simulink library "lib_flux_observer"  (R2023a)
settings: Solver=VariableStepAuto  StartTime=0.0  StopTime=10.0  RelTol=1e-3
undefined symbols (not defined in the file): bit, parDirIndc_u16p29b0, parFluxObsFiltCoef, parMedTaskSampTime_u16d6b0, parPhsCurrMaxVal, parPhsRstnMaxVal, parPhsVoltMaxVal, parPolePairNum_u8n0b0
libraries: lib_conversion x13, lib_trigonometric_function x2, lib_iir_filter x2, lib_discrete_time_integrator x2, lib_cart_to_polar_coor_transformer x1
settings Model: Creator=cav2ofo  LastModifiedBy=lenovo
settings OptimizationCC: ReuseModelBlockBuffer=off

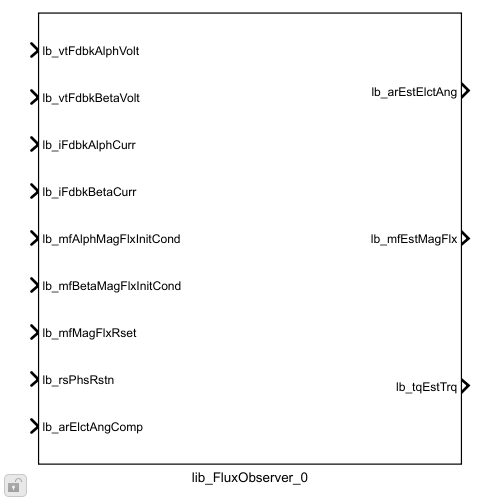
[thumbnail: Simulink's stored preview of the top-level diagram]
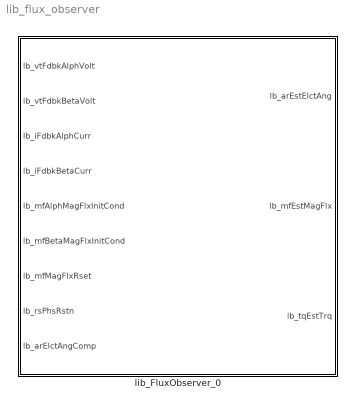
== system lib_flux_observer ==
  lib_FluxObserver_0 : Subsystem  mask{lb_parPhsIndc=parDirIndc_u16p29b0, lb_parPhsRstnMaxVal=parPhsRstnMaxVal, lb_parPhsIndcMaxVal=parPhsRstnMaxVal, lb_parPhsCurrMaxVal=parPhsCurrMaxVal, lb_parPhsVoltMaxVal=parPhsVoltMaxVal, lb_parEstMagFluxMaxVal=0.01, lb_parPolePairNum=parPolePairNum_u8n0b0, lb_parSampTime=parMedTaskSampTime_u16d6b0, lb_parFltrCoefMaxVal=double(parFluxObsFiltCoef), lb_parFiltCoef=parFluxObsFiltCoef, lb_parFluxDataType=fixdt(0,16,2^-22,0), lb_parMotTrqDataType=fixdt(1,16,2^-14,0), lb_parBitNumMode=32-bit}
      mask prompts: lb_parPhsIndc "Phase inductance [H]:"; lb_parPhsRstnMaxVal "Maximum phase resistance [Ohm]:"; lb_parPhsIndcMaxVal "Maximum phase inductance [H]:"; lb_parPhsCurrMaxVal "Maximum phase current [A]:"; lb_parPhsVoltMaxVal "Maximum phase voltage [V]:"; lb_parEstMagFluxMaxVal "Maximum estimated magnet flux [Wb]:"; lb_parPolePairNum "Number of pole pairs:"; lb_parSampTime "Sampling time [s]:"; lb_parFltrCoefMaxVal "High-pass filter coefficient max value:"; lb_parFiltCoef "High-pass filter coefficient:"; lb_parFluxDataType "Permanent magnet flux data type:"; lb_parMotTrqDataType "Motor electric torque data type:"; lb_parBitNumMode "Bits number for internal calculations:"
      mask init:
      | switch lb_parBitNumMode
      |     case '16-bit'
      |         lb_parBitNum = 16;
      |     case '32-bit'
      |         lb_parBitNum = 32;
      |     otherwise
      |         lb_parBitNum = 16;
      | end
      | 
      | % Operation 1: R*I
      | lb_parOper1MaxVal = lb_parPhsRstnMaxVal*lb_parPhsCurrMaxVal;
      | 
      | % Operation 2: V-R*I
      | lb_parOper2MaxVal = lb_parPhsVoltMaxVal+lb_parPhsRstnMaxVal*lb_parPhsCurrMaxVal;
      | 
      | % Operation 3: L*I
      | lb_parOper3MaxVal = lb_parPhsIndcMaxVal*lb_parPhsCurrMaxVal;
      | 
      | % Operation 4: integral of V-R*I
      | temp.intgMaxVal = lb_parOper3MaxVal+lb_parEstMagFluxMaxVal;
      | temp.NumType = fi(temp.intgMaxVal,1,lb_parBitNum);
      | lb_parIntgSlopExp = temp.NumType.FractionLength;
      | 
      | % Operation 5: filtering of flux
      | temp.NumType = fi(lb_parEstMagFluxMaxVal,1,16);
      | lb_parFiltSlopExp = temp.NumType.FractionLength;
      | 
      | % Operation 6: psi*I
      | lb_parOper6MaxVal = lb_parPhsCurrMaxVal*lb_parEstMagFluxMaxVal;
      | 
      | % Operation 7: 2*psi*I
      | lb_parOper7MaxVal = 2*lb_parPhsCurrMaxVal*lb_parEstMagFluxMaxVal;
      | 
      | % Operation 8: 3/2*Np
      | lb_parOper8MaxVal = 3/2*double(lb_parPolePairNum);
      mask TypeOptions lb_parFltrCoefMaxVal: sss_FluxAlphaBetaEstimation/lib_IirFilter_1/lb_parFltrCoefMaxVal | sss_FluxAlphaBetaEstimation/lib_IirFilter_2/lb_parFltrCoefMaxVal
      mask TypeOptions lb_parBitNumMode: 16-bit | 32-bit
      mask DialogControl DescGroupVar Prompt: Current Coupling block
      mask DialogControl DescTextVar Prompt: This block estimates electric angle, Permenant magnet flux and electric torque
      mask DialogControl modlPar Prompt: Model Parameters
      mask DialogControl Container3_copy Prompt: Data type:
      mask DialogControl Container3 Prompt: Operating modes:

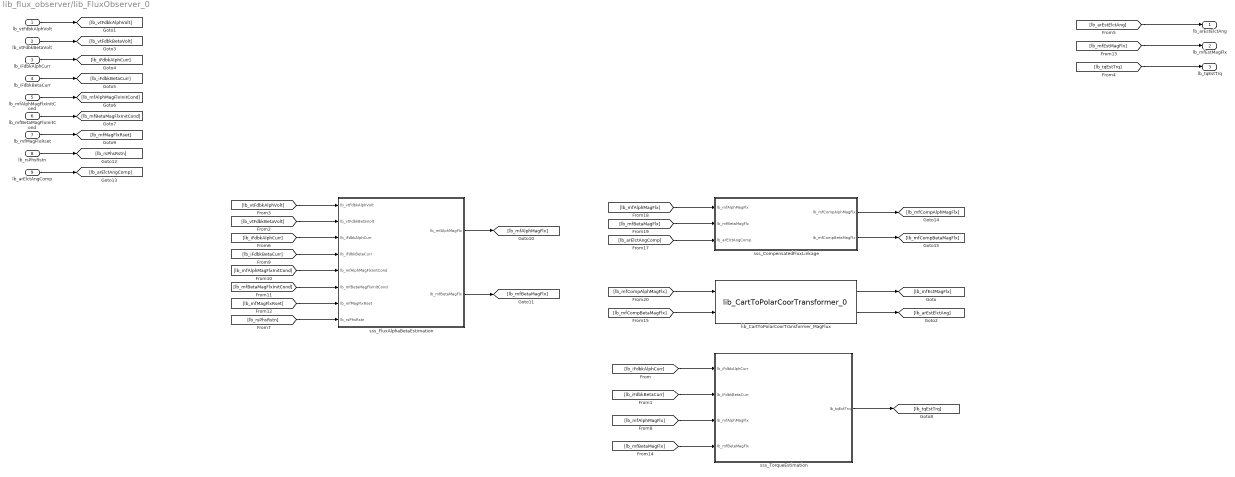
== system lib_flux_observer/lib_FluxObserver_0 ==
  lb_vtFdbkAlphVolt : Inport
  lb_vtFdbkBetaVolt : Inport  Port=2
  lb_iFdbkAlphCurr : Inport  Port=3
  lb_iFdbkBetaCurr : Inport  Port=4
  lb_mfAlphMagFlxInitCond : Inport  Port=5
  lb_mfBetaMagFlxInitCond : Inport  Port=6
  lb_mfMagFlxRset : Inport  Port=7
  lb_rsPhsRstn : Inport  Port=8
  lb_arElctAngComp : Inport  Port=9  OutDataTypeStr=fixdt(0,16,pi*2^-15,0)
  lib_CartToPolarCoorTransformer_MagFlux : lib_cart_to_polar_coor_transformer/lib_CartToPolarCoorTransformer_0  lb_parAsinLktSize=4095  lb_parAmpLktSize=512  lb_parOutpAmpDataType=lb_parFluxDataType
  sss_CompensatedFluxLinkage : Subsystem
  sss_FluxAlphaBetaEstimation : Subsystem
  sss_TorqueEstimation : Subsystem
  lb_arEstElctAng : Outport
  lb_mfEstMagFlx : Outport  Port=2
  lb_tqEstTrq : Outport  Port=3
  wires:
  sss_CompensatedFluxLinkage/2(lb_mfCompBetaMagFlx) -> [lb_mfCompBetaMagFlx]
  sss_CompensatedFluxLinkage/1(lb_mfCompAlphMagFlx) -> [lb_mfCompAlphMagFlx]
  [lb_mfBetaMagFlx] -> sss_CompensatedFluxLinkage/2(lb_mfBetaMagFlx)
  [lb_mfAlphMagFlx] -> sss_CompensatedFluxLinkage/1(lb_mfAlphMagFlx)
  [lb_arElctAngComp] -> sss_CompensatedFluxLinkage/3(lb_arElctAngComp)
  lb_arElctAngComp/1 -> [lb_arElctAngComp]
  [lb_rsPhsRstn] -> sss_FluxAlphaBetaEstimation/8(lb_rsPhsRstn)
  lb_rsPhsRstn/1 -> [lb_rsPhsRstn]
  [lb_mfCompAlphMagFlx] -> lib_CartToPolarCoorTransformer_MagFlux/1
  [lb_mfCompBetaMagFlx] -> lib_CartToPolarCoorTransformer_MagFlux/2
  lib_CartToPolarCoorTransformer_MagFlux/2 -> [lb_arEstElctAng]
  [lb_tqEstTrq] -> lb_tqEstTrq/1
  [lb_iFdbkBetaCurr] -> sss_TorqueEstimation/2(lb_iFdbkBetaCurr)
  [lb_iFdbkAlphCurr] -> sss_TorqueEstimation/1(lb_iFdbkAlphCurr)
  [lb_mfBetaMagFlx] -> sss_TorqueEstimation/4(lb_mfBetaMagFlx)
  [lb_mfAlphMagFlx] -> sss_TorqueEstimation/3(lb_mfAlphMagFlx)
  sss_FluxAlphaBetaEstimation/2(lb_mfBetaMagFlx) -> [lb_mfBetaMagFlx]
  sss_FluxAlphaBetaEstimation/1(lb_mfAlphMagFlx) -> [lb_mfAlphMagFlx]
  [lb_mfMagFlxRset] -> sss_FluxAlphaBetaEstimation/7(lb_mfMagFlxRset)
  lb_mfMagFlxRset/1 -> [lb_mfMagFlxRset]
  [lb_mfBetaMagFlxInitCond] -> sss_FluxAlphaBetaEstimation/6(lb_mfBetaMagFlxInitCond)
  [lb_mfAlphMagFlxInitCond] -> sss_FluxAlphaBetaEstimation/5(lb_mfAlphMagFlxInitCond)
  lb_mfAlphMagFlxInitCond/1 -> [lb_mfAlphMagFlxInitCond]
  lb_mfBetaMagFlxInitCond/1 -> [lb_mfBetaMagFlxInitCond]
  [lb_iFdbkBetaCurr] -> sss_FluxAlphaBetaEstimation/4(lb_iFdbkBetaCurr)
  [lb_vtFdbkBetaVolt] -> sss_FluxAlphaBetaEstimation/2(lb_vtFdbkBetaVolt)
  [lb_vtFdbkAlphVolt] -> sss_FluxAlphaBetaEstimation/1(lb_vtFdbkAlphVolt)
  lib_CartToPolarCoorTransformer_MagFlux/1 -> [lb_mfEstMagFlx]
  [lb_arEstElctAng] -> lb_arEstElctAng/1
  [lb_iFdbkAlphCurr] -> sss_FluxAlphaBetaEstimation/3(lb_iFdbkAlphCurr)
  lb_iFdbkAlphCurr/1 -> [lb_iFdbkAlphCurr]
  lb_vtFdbkBetaVolt/1 -> [lb_vtFdbkBetaVolt]
  sss_TorqueEstimation/1(lb_tqEstTrq) -> [lb_tqEstTrq]
  [lb_mfEstMagFlx] -> lb_mfEstMagFlx/1
  lb_iFdbkBetaCurr/1 -> [lb_iFdbkBetaCurr]
  lb_vtFdbkAlphVolt/1 -> [lb_vtFdbkAlphVolt]

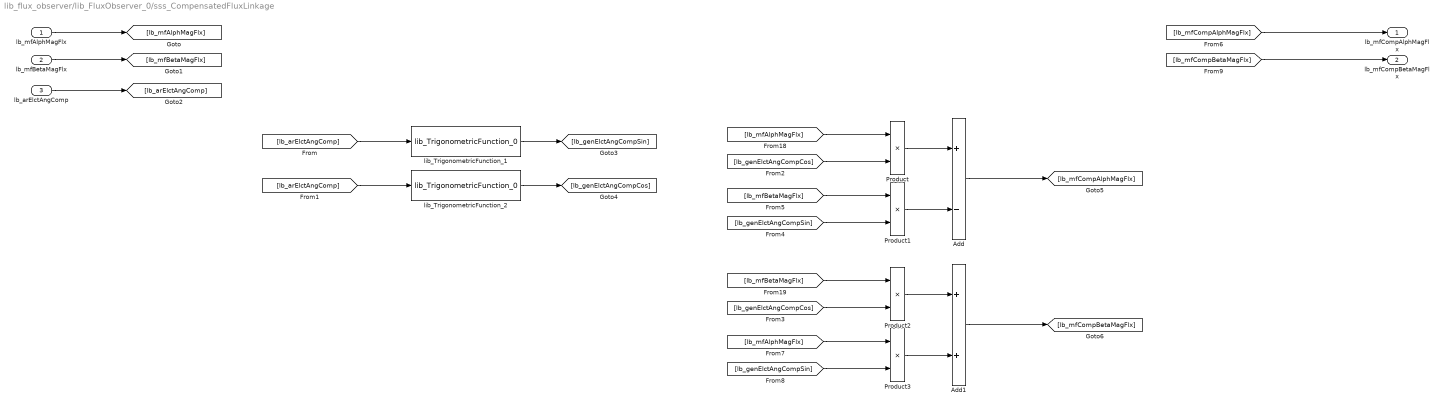
== system lib_flux_observer/lib_FluxObserver_0/sss_CompensatedFluxLinkage ==
  lb_mfAlphMagFlx : Inport
  lb_mfBetaMagFlx : Inport  Port=2
  lb_arElctAngComp : Inport  Port=3
  Add : Sum  Inputs=+-  OutDataTypeStr=Inherit: Same as first input
  Add1 : Sum  OutDataTypeStr=Inherit: Same as first input
  Product{,1..3} (4 alike) : Product  OutDataTypeStr=Inherit: Same as first input
  lib_TrigonometricFunction_1 : lib_trigonometric_function/lib_TrigonometricFunction_0  lb_parSelSigType=Sine  lb_parLktSizeStr=1024  lb_parOutpDataType=fixdt(1,16,2^-14,0)
  lib_TrigonometricFunction_2 : lib_trigonometric_function/lib_TrigonometricFunction_0  lb_parSelSigType=Cosine  lb_parLktSizeStr=1024  lb_parOutpDataType=fixdt(1,16,2^-14,0)
  lb_mfCompAlphMagFlx : Outport
  lb_mfCompBetaMagFlx : Outport  Port=2
  wires:
  [lb_mfCompBetaMagFlx] -> lb_mfCompBetaMagFlx/1
  [lb_mfCompAlphMagFlx] -> lb_mfCompAlphMagFlx/1
  Product2/1 -> Add1/1
  [lb_mfBetaMagFlx] -> Product2/1
  Product3/1 -> Add1/2
  Add1/1 -> [lb_mfCompBetaMagFlx]
  [lb_genElctAngCompSin] -> Product3/2
  [lb_genElctAngCompCos] -> Product2/2
  [lb_mfAlphMagFlx] -> Product3/1
  Add/1 -> [lb_mfCompAlphMagFlx]
  Product/1 -> Add/1
  Product1/1 -> Add/2
  [lb_mfBetaMagFlx] -> Product1/1
  [lb_genElctAngCompSin] -> Product1/2
  [lb_genElctAngCompCos] -> Product/2
  [lb_mfAlphMagFlx] -> Product/1
  lib_TrigonometricFunction_2/1 -> [lb_genElctAngCompCos]
  lib_TrigonometricFunction_1/1 -> [lb_genElctAngCompSin]
  [lb_arElctAngComp] -> lib_TrigonometricFunction_2/1
  [lb_arElctAngComp] -> lib_TrigonometricFunction_1/1
  lb_arElctAngComp/1 -> [lb_arElctAngComp]
  lb_mfBetaMagFlx/1 -> [lb_mfBetaMagFlx]
  lb_mfAlphMagFlx/1 -> [lb_mfAlphMagFlx]

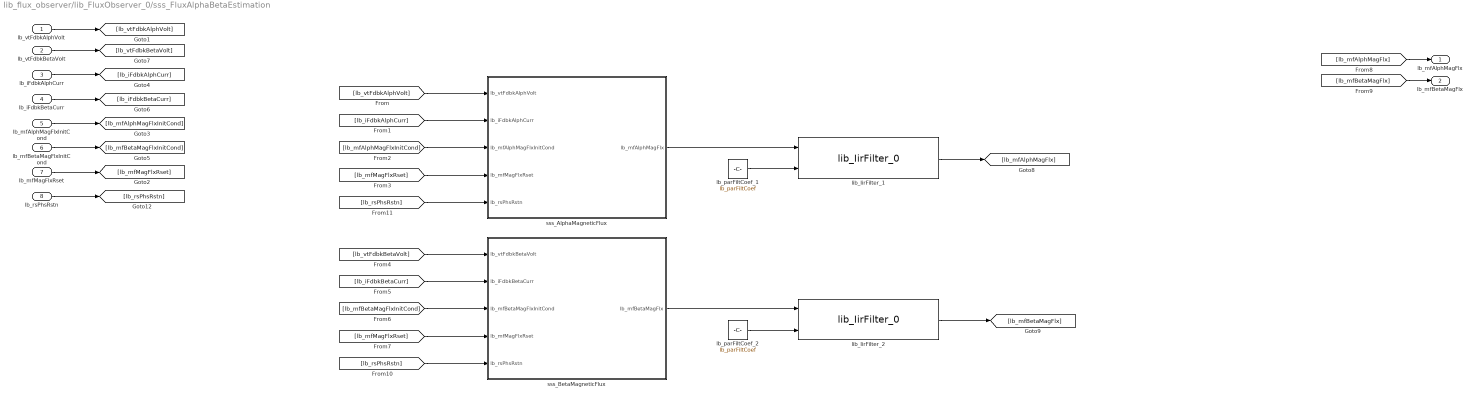
== system lib_flux_observer/lib_FluxObserver_0/sss_FluxAlphaBetaEstimation ==
  lb_vtFdbkAlphVolt : Inport
  lb_vtFdbkBetaVolt : Inport  Port=2
  lb_iFdbkAlphCurr : Inport  Port=3
  lb_iFdbkBetaCurr : Inport  Port=4
  lb_mfAlphMagFlxInitCond : Inport  Port=5
  lb_mfBetaMagFlxInitCond : Inport  Port=6
  lb_mfMagFlxRset : Inport  Port=7
  lb_rsPhsRstn : Inport  Port=8
  lb_parFiltCoef_1 : Constant  Value=lb_parFiltCoef
  lb_parFiltCoef_2 : Constant  Value=lb_parFiltCoef
  lib_IirFilter_1 : lib_iir_filter/lib_IirFilter_0  lb_parMaxInpVal=lb_parEstMagFluxMaxVal  lb_parFltrCoefMaxVal=lb_parFltrCoefMaxVal  lb_parBitNumMode=32-bit  lb_parOutpDataType=fixdt(1,16,2^-lb_parFiltSlopExp,0)  lb_parFiltTypeMode=High-pass
      link override vss_FilterVariant: VariantControlMode=label  LabelModeActiveChoice=lb_parHighPassModeLbl
  lib_IirFilter_2 : lib_iir_filter/lib_IirFilter_0  lb_parMaxInpVal=lb_parEstMagFluxMaxVal  lb_parFltrCoefMaxVal=lb_parFltrCoefMaxVal  lb_parBitNumMode=32-bit  lb_parOutpDataType=fixdt(1,16,2^-lb_parFiltSlopExp,0)  lb_parFiltTypeMode=High-pass
      link override vss_FilterVariant: VariantControlMode=label  LabelModeActiveChoice=lb_parHighPassModeLbl
  sss_AlphaMagneticFlux : Subsystem
  sss_BetaMagneticFlux : Subsystem
  lb_mfAlphMagFlx : Outport
  lb_mfBetaMagFlx : Outport  Port=2
  wires:
  lib_IirFilter_2/1 -> [lb_mfBetaMagFlx]
  lb_parFiltCoef_2/1 -> lib_IirFilter_2/2
  lb_parFiltCoef_1/1 -> lib_IirFilter_1/2
  sss_BetaMagneticFlux/1(lb_mfBetaMagFlx) -> lib_IirFilter_2/1
  [lb_rsPhsRstn] -> sss_AlphaMagneticFlux/5(lb_rsPhsRstn)
  [lb_rsPhsRstn] -> sss_BetaMagneticFlux/5(lb_rsPhsRstn)
  lb_rsPhsRstn/1 -> [lb_rsPhsRstn]
  lib_IirFilter_1/1 -> [lb_mfAlphMagFlx]
  sss_AlphaMagneticFlux/1(lb_mfAlphMagFlx) -> lib_IirFilter_1/1
  [lb_mfBetaMagFlx] -> lb_mfBetaMagFlx/1
  [lb_mfAlphMagFlx] -> lb_mfAlphMagFlx/1
  lb_vtFdbkBetaVolt/1 -> [lb_vtFdbkBetaVolt]
  lb_iFdbkBetaCurr/1 -> [lb_iFdbkBetaCurr]
  [lb_mfMagFlxRset] -> sss_BetaMagneticFlux/4(lb_mfMagFlxRset)
  [lb_vtFdbkBetaVolt] -> sss_BetaMagneticFlux/1(lb_vtFdbkBetaVolt)
  [lb_iFdbkBetaCurr] -> sss_BetaMagneticFlux/2(lb_iFdbkBetaCurr)
  [lb_mfBetaMagFlxInitCond] -> sss_BetaMagneticFlux/3(lb_mfBetaMagFlxInitCond)
  [lb_mfMagFlxRset] -> sss_AlphaMagneticFlux/4(lb_mfMagFlxRset)
  [lb_mfAlphMagFlxInitCond] -> sss_AlphaMagneticFlux/3(lb_mfAlphMagFlxInitCond)
  [lb_iFdbkAlphCurr] -> sss_AlphaMagneticFlux/2(lb_iFdbkAlphCurr)
  [lb_vtFdbkAlphVolt] -> sss_AlphaMagneticFlux/1(lb_vtFdbkAlphVolt)
  lb_mfBetaMagFlxInitCond/1 -> [lb_mfBetaMagFlxInitCond]
  lb_mfMagFlxRset/1 -> [lb_mfMagFlxRset]
  lb_vtFdbkAlphVolt/1 -> [lb_vtFdbkAlphVolt]
  lb_mfAlphMagFlxInitCond/1 -> [lb_mfAlphMagFlxInitCond]
  lb_iFdbkAlphCurr/1 -> [lb_iFdbkAlphCurr]

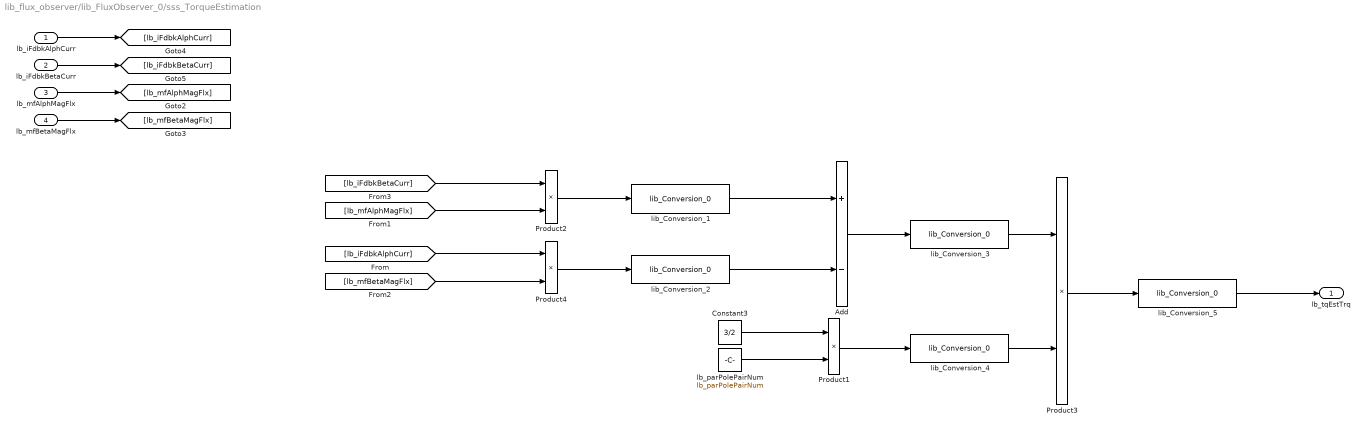
== system lib_flux_observer/lib_FluxObserver_0/sss_TorqueEstimation ==
  lb_iFdbkAlphCurr : Inport
  lb_iFdbkBetaCurr : Inport  Port=2
  lb_mfAlphMagFlx : Inport  Port=3
  lb_mfBetaMagFlx : Inport  Port=4
  Add : Sum  Inputs=+-  OutDataTypeStr=Inherit: Inherit via back propagation
  Constant3 : Constant  Value=3/2  OutDataTypeStr=fixdt(0,16,2^-15,0)
  Product{1..4} (4 alike) : Product  OutDataTypeStr=Inherit: Inherit via back propagation
  lb_parPolePairNum : Constant  Value=lb_parPolePairNum
  lib_Conversion_1 : lib_conversion/lib_Conversion_0  lb_parDataType=fixdt(1,16)  lb_parOutpMaxVal=lb_parOper6MaxVal  lb_parOutpMinVal=-lb_parOper6MaxVal  lb_parSatFlag=off
  lib_Conversion_2 : lib_conversion/lib_Conversion_0  lb_parDataType=fixdt(1,16)  lb_parOutpMaxVal=lb_parOper6MaxVal  lb_parOutpMinVal=-lb_parOper6MaxVal  lb_parSatFlag=off
  lib_Conversion_3 : lib_conversion/lib_Conversion_0  lb_parDataType=fixdt(1,16)  lb_parOutpMaxVal=lb_parOper7MaxVal  lb_parOutpMinVal=-lb_parOper7MaxVal  lb_parSatFlag=off
  lib_Conversion_4 : lib_conversion/lib_Conversion_0  lb_parDataType=fixdt(0,16)  lb_parOutpMaxVal=lb_parOper8MaxVal  lb_parOutpMinVal=[]  lb_parSatFlag=off
  lib_Conversion_5 : lib_conversion/lib_Conversion_0  lb_parDataType=lb_parMotTrqDataType  lb_parOutpMaxVal=[]  lb_parOutpMinVal=[]  lb_parSatFlag=off
  lb_tqEstTrq : Outport
  wires:
  lib_Conversion_2/1 -> Add/2
  Product4/1 -> lib_Conversion_2/1
  lib_Conversion_3/1 -> Product3/1
  lib_Conversion_4/1 -> Product3/2
  Product2/1 -> lib_Conversion_1/1
  lib_Conversion_1/1 -> Add/1
  Product1/1 -> lib_Conversion_4/1
  [lb_iFdbkBetaCurr] -> Product2/1
  [lb_mfAlphMagFlx] -> Product2/2
  [lb_iFdbkAlphCurr] -> Product4/1
  lb_iFdbkBetaCurr/1 -> [lb_iFdbkBetaCurr]
  lb_iFdbkAlphCurr/1 -> [lb_iFdbkAlphCurr]
  lb_parPolePairNum/1 -> Product1/2
  Constant3/1 -> Product1/1
  Add/1 -> lib_Conversion_3/1
  [lb_mfBetaMagFlx] -> Product4/2
  lib_Conversion_5/1 -> lb_tqEstTrq/1
  lb_mfBetaMagFlx/1 -> [lb_mfBetaMagFlx]
  lb_mfAlphMagFlx/1 -> [lb_mfAlphMagFlx]
  Product3/1 -> lib_Conversion_5/1

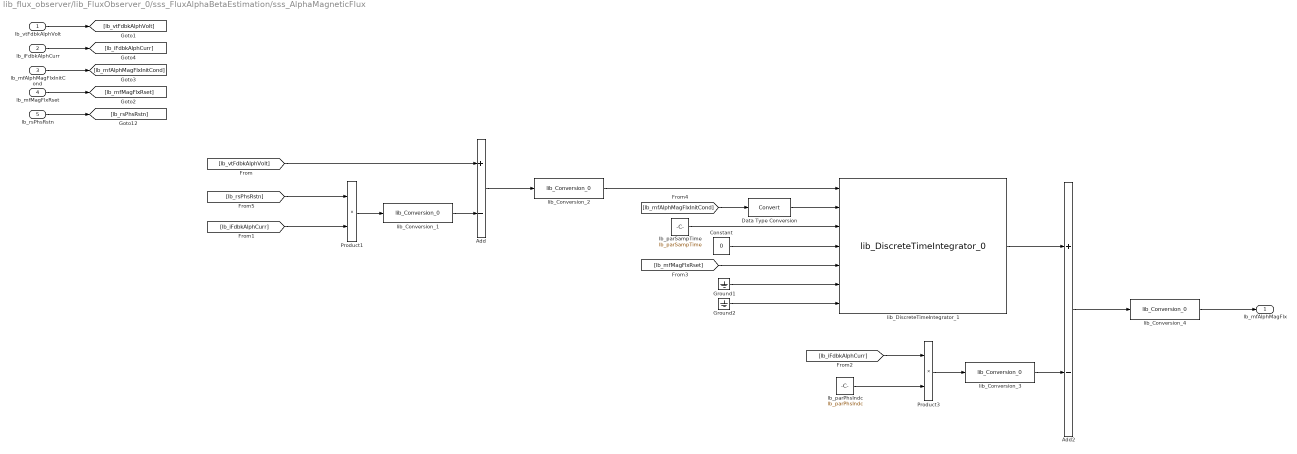
== system lib_flux_observer/lib_FluxObserver_0/sss_FluxAlphaBetaEstimation/sss_AlphaMagneticFlux ==
  lb_vtFdbkAlphVolt : Inport
  lb_iFdbkAlphCurr : Inport  Port=2
  lb_mfAlphMagFlxInitCond : Inport  Port=3
  lb_mfMagFlxRset : Inport  Port=4
  lb_rsPhsRstn : Inport  Port=5
  Add : Sum  Inputs=+-  OutDataTypeStr=Inherit: Inherit via back propagation
  Add2 : Sum  Inputs=+-  OutDataTypeStr=Inherit: Inherit via back propagation
  Constant : Constant  Value=0  OutDataTypeStr=uint8
  Data Type Conversion : DataTypeConversion  SaturateOnIntegerOverflow=off  RndMeth=Floor
  Ground1 : Ground
  Ground2 : Ground
  Product1 : Product  OutDataTypeStr=Inherit: Inherit via back propagation
  Product3 : Product  OutDataTypeStr=Inherit: Inherit via back propagation
  lb_parPhsIndc : Constant  Value=lb_parPhsIndc
  lb_parSampTime : Constant  Value=lb_parSampTime
  lib_Conversion_1 : lib_conversion/lib_Conversion_0  lb_parDataType=fixdt(1,lb_parBitNum)  lb_parOutpMaxVal=lb_parOper1MaxVal  lb_parOutpMinVal=-lb_parOper1MaxVal  lb_parSatFlag=off
  lib_Conversion_2 : lib_conversion/lib_Conversion_0  lb_parDataType=fixdt(1,lb_parBitNum)  lb_parOutpMaxVal=lb_parOper2MaxVal  lb_parOutpMinVal=-lb_parOper2MaxVal  lb_parSatFlag=off
  lib_Conversion_3 : lib_conversion/lib_Conversion_0  lb_parDataType=fixdt(1,lb_parBitNum)  lb_parOutpMaxVal=lb_parOper3MaxVal  lb_parOutpMinVal=-lb_parOper3MaxVal  lb_parSatFlag=off
  lib_Conversion_4 : lib_conversion/lib_Conversion_0  lb_parDataType=fixdt(1,lb_parBitNum)  lb_parOutpMaxVal=lb_parEstMagFluxMaxVal  lb_parOutpMinVal=-lb_parEstMagFluxMaxVal  lb_parSatFlag=off
  lib_DiscreteTimeIntegrator_1 : lib_discrete_time_integrator/lib_DiscreteTimeIntegrator_0  lb_parMaxInpVal=lb_parOper2MaxVal  lb_parMinInpVal=-lb_parOper2MaxVal  lb_parMaxSampTime=double(lb_parSampTime)  lb_parMaxIntgGain=0  lb_parAccmDataTypeMode=32-bit  lb_parOutpDataType=fixdt(1,lb_parBitNum,2^-lb_parIntgSlopExp,0)  lb_parIntgScopMode=Generic signal  lb_parSatFlag=off
  lb_mfAlphMagFlx : Outport
  wires:
  Data Type Conversion/1 -> lib_DiscreteTimeIntegrator_1/2
  [lb_iFdbkAlphCurr] -> Product3/1
  Product3/1 -> lib_Conversion_3/1
  lib_Conversion_3/1 -> Add2/2
  lib_DiscreteTimeIntegrator_1/1 -> Add2/1
  Add2/1 -> lib_Conversion_4/1
  lb_parPhsIndc/1 -> Product3/2
  lb_rsPhsRstn/1 -> [lb_rsPhsRstn]
  lib_Conversion_1/1 -> Add/2
  [lb_mfMagFlxRset] -> lib_DiscreteTimeIntegrator_1/5
  Constant/1 -> lib_DiscreteTimeIntegrator_1/4
  Ground2/1 -> lib_DiscreteTimeIntegrator_1/7
  lib_Conversion_2/1 -> lib_DiscreteTimeIntegrator_1/1
  lb_parSampTime/1 -> lib_DiscreteTimeIntegrator_1/3
  Ground1/1 -> lib_DiscreteTimeIntegrator_1/6
  lib_Conversion_4/1 -> lb_mfAlphMagFlx/1
  Product1/1 -> lib_Conversion_1/1
  lb_mfMagFlxRset/1 -> [lb_mfMagFlxRset]
  lb_vtFdbkAlphVolt/1 -> [lb_vtFdbkAlphVolt]
  lb_iFdbkAlphCurr/1 -> [lb_iFdbkAlphCurr]
  lb_mfAlphMagFlxInitCond/1 -> [lb_mfAlphMagFlxInitCond]
  [lb_vtFdbkAlphVolt] -> Add/1
  [lb_iFdbkAlphCurr] -> Product1/2
  [lb_rsPhsRstn] -> Product1/1
  [lb_mfAlphMagFlxInitCond] -> Data Type Conversion/1
  Add/1 -> lib_Conversion_2/1

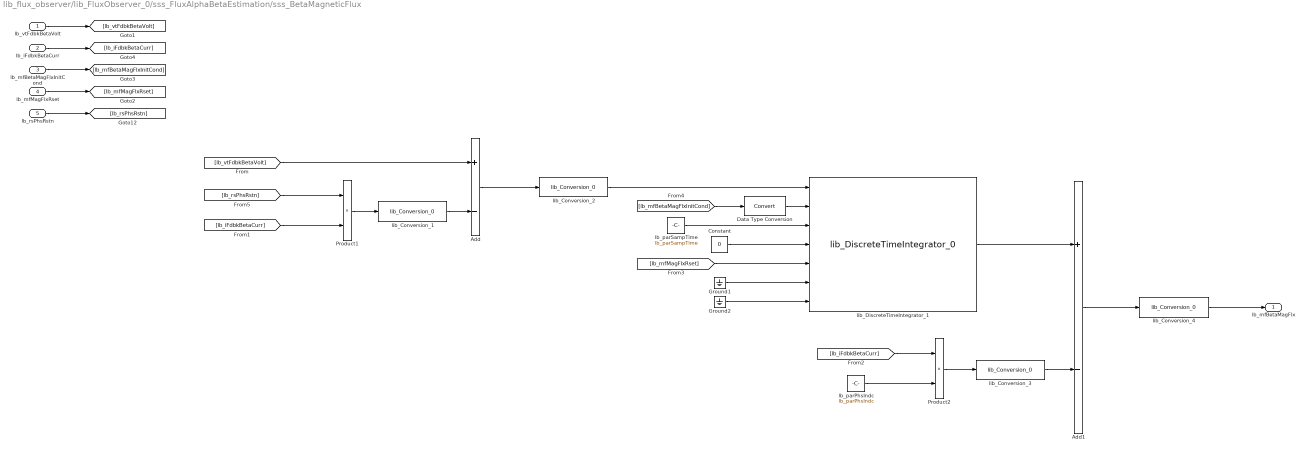
== system lib_flux_observer/lib_FluxObserver_0/sss_FluxAlphaBetaEstimation/sss_BetaMagneticFlux ==
  lb_vtFdbkBetaVolt : Inport
  lb_iFdbkBetaCurr : Inport  Port=2
  lb_mfBetaMagFlxInitCond : Inport  Port=3
  lb_mfMagFlxRset : Inport  Port=4
  lb_rsPhsRstn : Inport  Port=5
  Add : Sum  Inputs=+-  OutDataTypeStr=Inherit: Inherit via back propagation
  Add1 : Sum  Inputs=+-  OutDataTypeStr=Inherit: Inherit via back propagation
  Constant : Constant  Value=0  OutDataTypeStr=uint8
  Data Type Conversion : DataTypeConversion  SaturateOnIntegerOverflow=off  RndMeth=Floor
  Ground1 : Ground
  Ground2 : Ground
  Product1 : Product  OutDataTypeStr=Inherit: Inherit via back propagation
  Product2 : Product  OutDataTypeStr=Inherit: Inherit via back propagation
  lb_parPhsIndc : Constant  Value=lb_parPhsIndc
  lb_parSampTime : Constant  Value=lb_parSampTime
  lib_Conversion_1 : lib_conversion/lib_Conversion_0  lb_parDataType=fixdt(1,lb_parBitNum)  lb_parOutpMaxVal=lb_parOper1MaxVal  lb_parOutpMinVal=-lb_parOper1MaxVal  lb_parSatFlag=off
  lib_Conversion_2 : lib_conversion/lib_Conversion_0  lb_parDataType=fixdt(1,lb_parBitNum)  lb_parOutpMaxVal=lb_parOper2MaxVal  lb_parOutpMinVal=-lb_parOper2MaxVal  lb_parSatFlag=off
  lib_Conversion_3 : lib_conversion/lib_Conversion_0  lb_parDataType=fixdt(1,lb_parBitNum)  lb_parOutpMaxVal=lb_parOper3MaxVal  lb_parOutpMinVal=-lb_parOper3MaxVal  lb_parSatFlag=off
  lib_Conversion_4 : lib_conversion/lib_Conversion_0  lb_parDataType=fixdt(1,lb_parBitNum)  lb_parOutpMaxVal=lb_parEstMagFluxMaxVal  lb_parOutpMinVal=-lb_parEstMagFluxMaxVal  lb_parSatFlag=off
  lib_DiscreteTimeIntegrator_1 : lib_discrete_time_integrator/lib_DiscreteTimeIntegrator_0  lb_parMaxInpVal=lb_parOper2MaxVal  lb_parMinInpVal=-lb_parOper2MaxVal  lb_parMaxSampTime=double(lb_parSampTime)  lb_parMaxIntgGain=0  lb_parAccmDataTypeMode=32-bit  lb_parOutpDataType=fixdt(1,lb_parBitNum,2^-lb_parIntgSlopExp,0)  lb_parIntgScopMode=Generic signal  lb_parSatFlag=off
  lb_mfBetaMagFlx : Outport
  wires:
  Data Type Conversion/1 -> lib_DiscreteTimeIntegrator_1/2
  lib_Conversion_3/1 -> Add1/2
  Ground2/1 -> lib_DiscreteTimeIntegrator_1/7
  Constant/1 -> lib_DiscreteTimeIntegrator_1/4
  [lb_mfMagFlxRset] -> lib_DiscreteTimeIntegrator_1/5
  Ground1/1 -> lib_DiscreteTimeIntegrator_1/6
  lb_parSampTime/1 -> lib_DiscreteTimeIntegrator_1/3
  [lb_mfBetaMagFlxInitCond] -> Data Type Conversion/1
  lib_Conversion_2/1 -> lib_DiscreteTimeIntegrator_1/1
  lib_Conversion_1/1 -> Add/2
  lb_rsPhsRstn/1 -> [lb_rsPhsRstn]
  lib_Conversion_4/1 -> lb_mfBetaMagFlx/1
  Product1/1 -> lib_Conversion_1/1
  Add/1 -> lib_Conversion_2/1
  [lb_vtFdbkBetaVolt] -> Add/1
  lb_mfMagFlxRset/1 -> [lb_mfMagFlxRset]
  lb_vtFdbkBetaVolt/1 -> [lb_vtFdbkBetaVolt]
  lb_iFdbkBetaCurr/1 -> [lb_iFdbkBetaCurr]
  lb_mfBetaMagFlxInitCond/1 -> [lb_mfBetaMagFlxInitCond]
  [lb_iFdbkBetaCurr] -> Product1/2
  lb_parPhsIndc/1 -> Product2/2
  [lb_rsPhsRstn] -> Product1/1
  lib_DiscreteTimeIntegrator_1/1 -> Add1/1
  [lb_iFdbkBetaCurr] -> Product2/1
  Product2/1 -> lib_Conversion_3/1
  Add1/1 -> lib_Conversion_4/1
